simulink model "RobotR2018a"  (R2018a)
settings: Solver=FixedStepAuto  StartTime=0.0  StopTime=200  FixedStep=0.01  RelTol=1e-3  EnableMultiTasking=on
libraries: arduinolib x12
settings Model: ExtModeTrigDuration=2  Creator=SINA  LastModifiedBy=SINA
settings SolverCC: AutoInsertRateTranBlk=on
settings DataIOCC: ReturnWorkspaceOutputs=on
settings OptimizationCC: EnhancedBackFolding=on  PassReuseOutputArgsAs=Individual arguments  ZeroExternalMemoryAtStartup=off  ZeroInternalMemoryAtStartup=off  MaxStackSize=64  OptimizeBlockOrder=speed  DifferentSizesBufferReuse=on  OptimizationCustomize=off
settings DebuggingCC: ParameterTunabilityLossMsg=error  UnconnectedInputMsg=none  UnconnectedOutputMsg=none  UnconnectedLineMsg=none  SFMachineParentedDataDiag=error
settings HardwareCC: ProdBitPerInt=16  ProdBitPerPointer=16  ProdBitPerSizeT=16  ProdBitPerPtrDiffT=16  ProdLargestAtomicFloat=None  ProdWordSize=8  ProdHWDeviceType=Atmel->AVR
settings SFSimCC: SimUseLocalCustomCode=on  MATLABDynamicMemAlloc=off
settings RTWCC: SystemTargetFile=ert.tlc  HardwareBoard=Arduino Uno  TLCOptions=-aInlineSetEventsForThisBaseRateFcn=TLC_FALSE -aSuppressMultiTaskScheduler=TLC_FALSE -aRateBasedStepFcn=1  TemplateMakefile=ert_default_tmf  RTWUseLocalCustomCode=on  Toolchain=Arduino AVR  BuildConfiguration=Faster Runs
settings CodeAppCC: ForceParamTrailComments=on  IgnoreCustomStorageClasses=off  OperatorAnnotations=on  SimulinkDataObjDesc=on  SFDataObjDesc=on  InsertBlockDesc=on
settings ERTTargetCC: SupportContinuousTime=on  SupportVariableSizeSignals=on  ExtModeTransport=3  ExtModeStaticAlloc=on  ExtModeStaticAllocSize=250  ExtModeMexFile=ext_xcp  ExtModeIntrfLevel=Level2 - Open

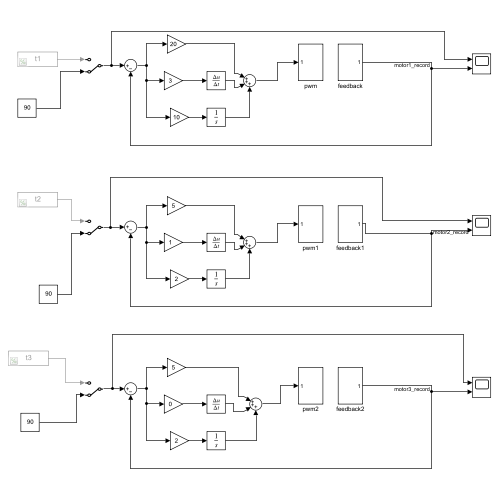
[thumbnail: Simulink's stored preview of the top-level diagram]
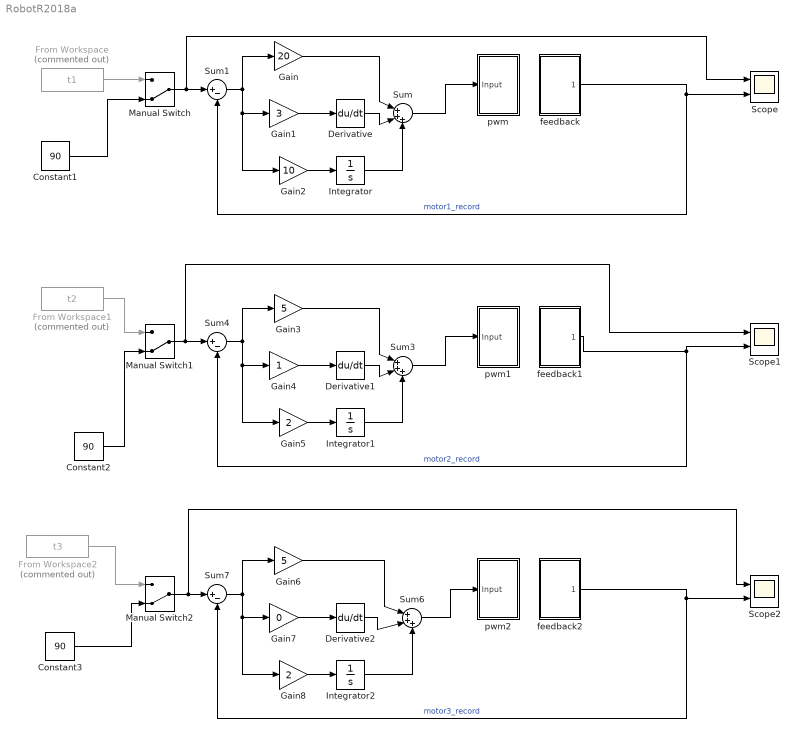
== system RobotR2018a ==
  Constant1 : Constant  Value=90
  Constant2 : Constant  Value=90
  Constant3 : Constant  Value=90
  Derivative : Derivative  CoefficientInTFapproximation=20
  Derivative1 : Derivative  CoefficientInTFapproximation=20
  Derivative2 : Derivative  CoefficientInTFapproximation=20
  From Workspace : FromWorkspace  Commented=on  VariableName=t1  SampleTime=0.2  Interpolate=off  OutputAfterFinalValue=Cyclic repetition
  From Workspace1 : FromWorkspace  Commented=on  VariableName=t2  SampleTime=0.2  Interpolate=off  OutputAfterFinalValue=Cyclic repetition
  From Workspace2 : FromWorkspace  Commented=on  VariableName=t3  SampleTime=0.2  Interpolate=off  OutputAfterFinalValue=Cyclic repetition
  Gain : Gain  Gain=20
  Gain1 : Gain  Gain=3
  Gain2 : Gain  Gain=10
  Gain3 : Gain  Gain=5
  Gain4 : Gain
  Gain5 : Gain  Gain=2
  Gain6 : Gain  Gain=5
  Gain7 : Gain  Gain=0
  Gain8 : Gain  Gain=2
  Integrator : Integrator
  Integrator1 : Integrator
  Integrator2 : Integrator
  Manual Switch : ManualSwitch  CurrentSetting=0
  Manual Switch1 : ManualSwitch  CurrentSetting=0
  Manual Switch2 : ManualSwitch  CurrentSetting=0
  Scope : Scope  NumInputPorts=2
  Scope1 : Scope  NumInputPorts=2
  Scope2 : Scope  NumInputPorts=2
  Sum : Sum  Inputs=|+++
  Sum1 : Sum  Inputs=|+-
  Sum3 : Sum  Inputs=|+++
  Sum4 : Sum  Inputs=|+-
  Sum6 : Sum  Inputs=|+++
  Sum7 : Sum  Inputs=|+-
  feedback : Subsystem
  feedback1 : Subsystem
  feedback2 : Subsystem
  pwm : Subsystem
  pwm1 : Subsystem
  pwm2 : Subsystem
  wires:
  feedback/1(Output) -> Sum1/2, Scope/2  "motor1_record"
  Sum1/1 -> Gain/1, Gain2/1, Gain1/1
  Gain/1 -> Sum/1
  Derivative/1 -> Sum/2
  Integrator/1 -> Sum/3
  Gain1/1 -> Derivative/1
  Gain2/1 -> Integrator/1
  Manual Switch/1 -> Scope/1, Sum1/1
  From Workspace1/1 -> Manual Switch1/1
  Integrator1/1 -> Sum3/3
  Gain4/1 -> Derivative1/1
  Gain5/1 -> Integrator1/1
  Sum4/1 -> Gain3/1, Gain5/1, Gain4/1
  Manual Switch1/1 -> Scope1/1, Sum4/1
  feedback1/1(Output) -> Scope1/2, Sum4/2  "motor2_record"
  Derivative1/1 -> Sum3/2
  Gain3/1 -> Sum3/1
  Constant2/1 -> Manual Switch1/2
  Constant3/1 -> Manual Switch2/2
  Gain6/1 -> Sum6/1
  Integrator2/1 -> Sum6/3
  Sum7/1 -> Gain6/1, Gain8/1, Gain7/1
  Derivative2/1 -> Sum6/2
  feedback2/1(Output) -> Sum7/2, Scope2/2  "motor3_record"
  Gain7/1 -> Derivative2/1
  Gain8/1 -> Integrator2/1
  From Workspace2/1 -> Manual Switch2/1
  Manual Switch2/1 -> Scope2/1, Sum7/1
  From Workspace/1 -> Manual Switch/1
  Constant1/1 -> Manual Switch/2
  Sum/1 -> pwm/1(Input)
  Sum3/1 -> pwm1/1(Input)
  Sum6/1 -> pwm2/1(Input)

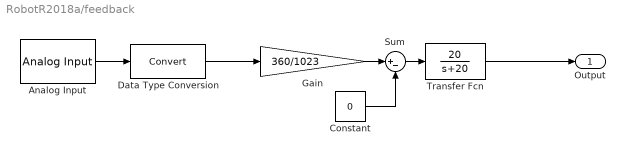
== system RobotR2018a/feedback ==
  Analog Input : arduinolib/Analog Input  pinNumber=1  ReadResultsOnly=off  ConversionTriggerSource=Software  ExternalTriggerType=uint32( 0 )  OutputDataType=uint16  EnableConversionCompleteNotify=off  EnableOuputStatus=off  SampleTime=0.01  blockPlatform=arduino
  Constant : Constant  Value=0
  Data Type Conversion : DataTypeConversion
  Gain : Gain  Gain=360/1023
  Sum : Sum  Inputs=|+-
  Transfer Fcn : TransferFcn  Numerator=[20]  Denominator=[1 20]
  Output : Outport
  wires:
  Analog Input/1 -> Data Type Conversion/1
  Data Type Conversion/1 -> Gain/1
  Transfer Fcn/1 -> Output/1
  Gain/1 -> Sum/1
  Sum/1 -> Transfer Fcn/1
  Constant/1 -> Sum/2

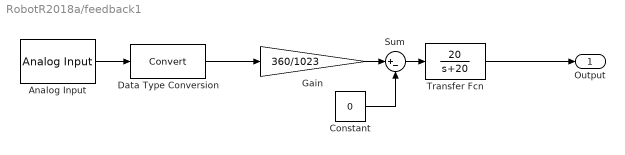
== system RobotR2018a/feedback1 ==
  Analog Input : arduinolib/Analog Input  pinNumber=2  ReadResultsOnly=off  ConversionTriggerSource=Software  ExternalTriggerType=uint32( 0 )  OutputDataType=uint16  EnableConversionCompleteNotify=off  EnableOuputStatus=off  SampleTime=0.01  blockPlatform=arduino
  Constant : Constant  Value=0
  Data Type Conversion : DataTypeConversion
  Gain : Gain  Gain=360/1023
  Sum : Sum  Inputs=|+-
  Transfer Fcn : TransferFcn  Numerator=[20]  Denominator=[1 20]
  Output : Outport
  wires:
  Analog Input/1 -> Data Type Conversion/1
  Data Type Conversion/1 -> Gain/1
  Transfer Fcn/1 -> Output/1
  Gain/1 -> Sum/1
  Sum/1 -> Transfer Fcn/1
  Constant/1 -> Sum/2

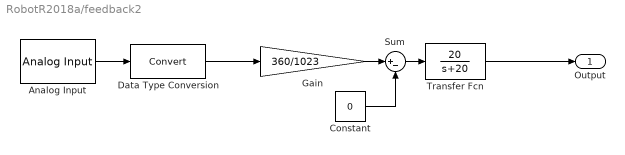
== system RobotR2018a/feedback2 ==
  Analog Input : arduinolib/Analog Input  pinNumber=3  ReadResultsOnly=off  ConversionTriggerSource=Software  ExternalTriggerType=uint32( 0 )  OutputDataType=uint16  EnableConversionCompleteNotify=off  EnableOuputStatus=off  SampleTime=0.01  blockPlatform=arduino
  Constant : Constant  Value=0
  Data Type Conversion : DataTypeConversion
  Gain : Gain  Gain=360/1023
  Sum : Sum  Inputs=|+-
  Transfer Fcn : TransferFcn  Numerator=[20]  Denominator=[1 20]
  Output : Outport
  wires:
  Analog Input/1 -> Data Type Conversion/1
  Data Type Conversion/1 -> Gain/1
  Transfer Fcn/1 -> Output/1
  Gain/1 -> Sum/1
  Sum/1 -> Transfer Fcn/1
  Constant/1 -> Sum/2

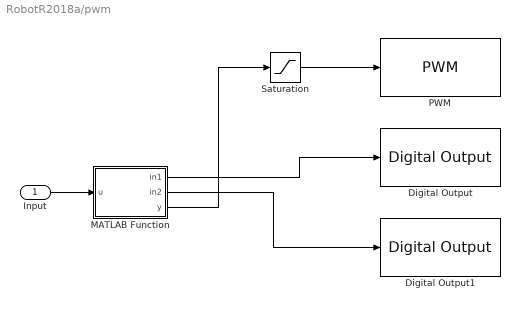
== system RobotR2018a/pwm ==
  Input : Inport
  Digital Output : arduinolib/Digital Output  pinNumber=7  Direction=output  blockPlatform=arduino
  Digital Output1 : arduinolib/Digital Output  pinNumber=8  Direction=output  blockPlatform=arduino
  MATLAB Function : MATLAB Function  TreatAsAtomicUnit=on
  PWM : arduinolib/PWM  pinNumber=6  frequencyType=Default  desiredFrequency=490.2  achievableFrequency=490.2
  Saturation : Saturate  UpperLimit=8/12*255  LowerLimit=0
  wires:
  MATLAB Function/2(in2) -> Digital Output1/1
  MATLAB Function/3(y) -> Saturation/1
  Saturation/1 -> PWM/1
  MATLAB Function/1(in1) -> Digital Output/1
  Input/1 -> MATLAB Function/1(u)

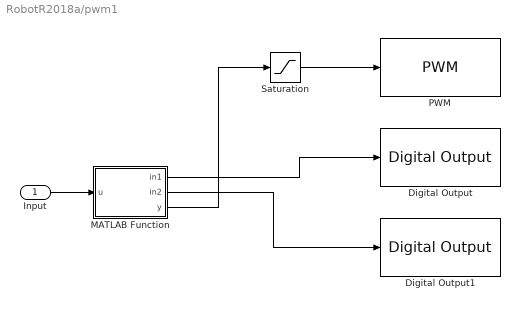
== system RobotR2018a/pwm1 ==
  Input : Inport
  Digital Output : arduinolib/Digital Output  pinNumber=2  Direction=output  blockPlatform=arduino
  Digital Output1 : arduinolib/Digital Output  pinNumber=4  Direction=output  blockPlatform=arduino
  MATLAB Function : MATLAB Function  TreatAsAtomicUnit=on
  PWM : arduinolib/PWM  pinNumber=3  frequencyType=Default  desiredFrequency=490.2  achievableFrequency=490.2
  Saturation : Saturate  UpperLimit=8/12*255  LowerLimit=0
  wires:
  MATLAB Function/2(in2) -> Digital Output1/1
  MATLAB Function/3(y) -> Saturation/1
  Saturation/1 -> PWM/1
  MATLAB Function/1(in1) -> Digital Output/1
  Input/1 -> MATLAB Function/1(u)

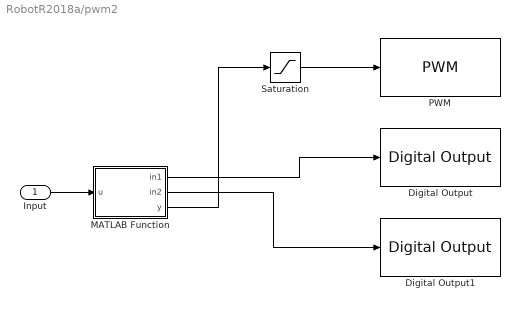
== system RobotR2018a/pwm2 ==
  Input : Inport
  Digital Output : arduinolib/Digital Output  pinNumber=12  Direction=output  blockPlatform=arduino
  Digital Output1 : arduinolib/Digital Output  pinNumber=13  Direction=output  blockPlatform=arduino
  MATLAB Function : MATLAB Function  TreatAsAtomicUnit=on
  PWM : arduinolib/PWM  pinNumber=11  frequencyType=Default  desiredFrequency=490.2  achievableFrequency=490.2
  Saturation : Saturate  UpperLimit=8/12*255  LowerLimit=0
  wires:
  MATLAB Function/2(in2) -> Digital Output1/1
  MATLAB Function/3(y) -> Saturation/1
  Saturation/1 -> PWM/1
  MATLAB Function/1(in1) -> Digital Output/1
  Input/1 -> MATLAB Function/1(u)

== matlab function RobotR2018a/pwm1/MATLAB Function ==
  data: in1 output; in2 output; u input; y output
function [in1,in2,y] = fcn(u)
if u > 0
    in1 = 0;
    in2 = 1;
    y=u;
else
    in1 = 1;
    in2 = 0;
    y = -u;
end

end

== matlab function RobotR2018a/pwm/MATLAB Function ==
  data: in1 output; in2 output; u input; y output
function [in1,in2,y] = fcn(u)
if u > 0
    in1 = 1;
    in2 = 0;
    y=u;
else
    in1 = 0;
    in2 = 1;
    y = -u;
end

end

== matlab function RobotR2018a/pwm2/MATLAB Function ==
  data: in1 output; in2 output; u input; y output
function [in1,in2,y] = fcn(u)
if u > 0
    in1 = 1;
    in2 = 0;
    y=u;
else
    in1 = 0;
    in2 = 1;
    y = -u;
end

end
